simulink model "hpf"  (R2020a)
settings: Solver=VariableStepAuto  StartTime=0.0  StopTime=10.0  RelTol=1e-3
model workspace (MAT data in the model file):
  A = Simulink.Parameter
  A.Value = 0.5792
  A.DataType = 'auto'
  A.Dimensions = [1 1]
  B = Simulink.Parameter
  B.Value = 0.1584
  B.DataType = 'auto'
  B.Dimensions = [1 1]
settings Model: Creator=akhil singh  LastModifiedBy=akhil singh

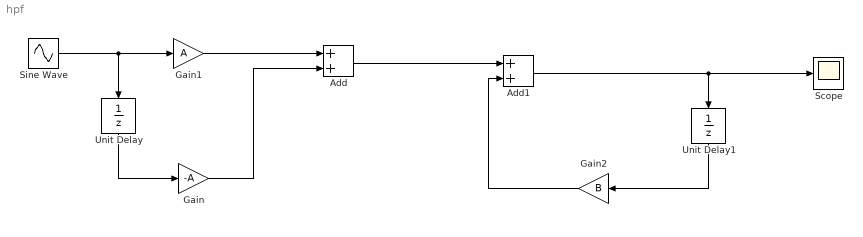
== system hpf ==
  Add : Sum
  Add1 : Sum
  Gain : Gain  Gain=-A
  Gain1 : Gain  Gain=A
  Gain2 : Gain  Gain=B
  Scope : Scope
  Sine Wave : Sin  SampleTime=0
  Unit Delay : UnitDelay  SampleTime=-1  HasFrameUpgradeWarning=on
  Unit Delay1 : UnitDelay  SampleTime=-1  HasFrameUpgradeWarning=on
  wires:
  Gain1/1 -> Add/1
  Gain/1 -> Add/2
  Gain2/1 -> Add1/2
  Add/1 -> Add1/1
  Unit Delay/1 -> Gain/1
  Sine Wave/1 -> Unit Delay/1, Gain1/1
  Unit Delay1/1 -> Gain2/1
  Add1/1 -> Unit Delay1/1, Scope/1
